simulink model "problem3"  (R2020b)
settings: Solver=VariableStepAuto  StartTime=0.0  StopTime=10.0  RelTol=1e-3
undefined symbols (not defined in the file): b, Ki, Kp, m
settings Model: Creator=Shivashis  LastModifiedBy=Shivashis

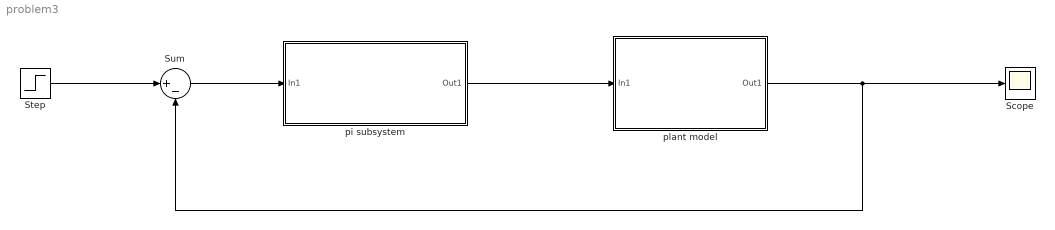
== system problem3 ==
  Scope : Scope
  Step : Step  SampleTime=0
  Sum : Sum  Inputs=|+-
  pi subsystem : Subsystem
  plant model : Subsystem
  wires:
  Step/1 -> Sum/1
  Sum/1 -> pi subsystem/1(In1)
  pi subsystem/1(Out1) -> plant model/1(In1)
  plant model/1(Out1) -> Sum/2, Scope/1

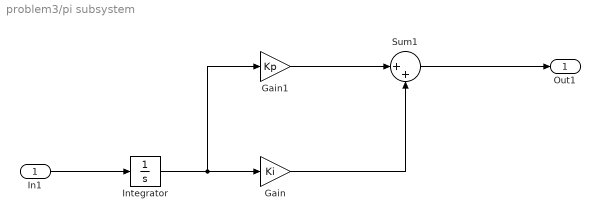
== system problem3/pi subsystem ==
  In1 : Inport
  Gain : Gain  Gain=Ki
  Gain1 : Gain  Gain=Kp
  Integrator : Integrator
  Sum1 : Sum  Inputs=|++
  Out1 : Outport
  wires:
  Sum1/1 -> Out1/1
  Gain/1 -> Sum1/2
  Gain1/1 -> Sum1/1
  In1/1 -> Integrator/1
  Integrator/1 -> Gain1/1, Gain/1

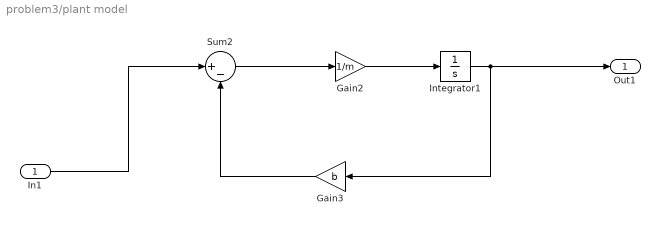
== system problem3/plant model ==
  In1 : Inport
  Gain2 : Gain  Gain=1/m
  Gain3 : Gain  Gain=b
  Integrator1 : Integrator
  Sum2 : Sum  Inputs=|+-
  Out1 : Outport
  wires:
  Gain2/1 -> Integrator1/1
  Gain3/1 -> Sum2/2
  Integrator1/1 -> Out1/1, Gain3/1
  In1/1 -> Sum2/1
  Sum2/1 -> Gain2/1
